simulink model "SimpleTurbine"  (R2023b)
settings: Solver=VariableStepAuto  StartTime=0.0  StopTime=10.0  RelTol=1e-3
undefined symbols (not defined in the file): A_VGS, cp, kap, N, p_in, p_out, R, RH_in, T_in
settings Model: Creator=KOTA-Z  LastModifiedBy=KOTA-Z

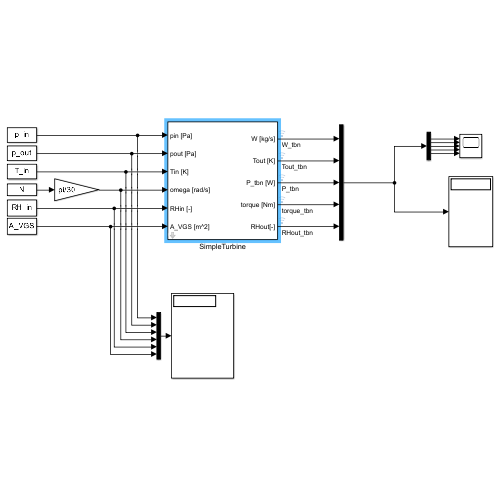
[thumbnail: Simulink's stored preview of the top-level diagram]
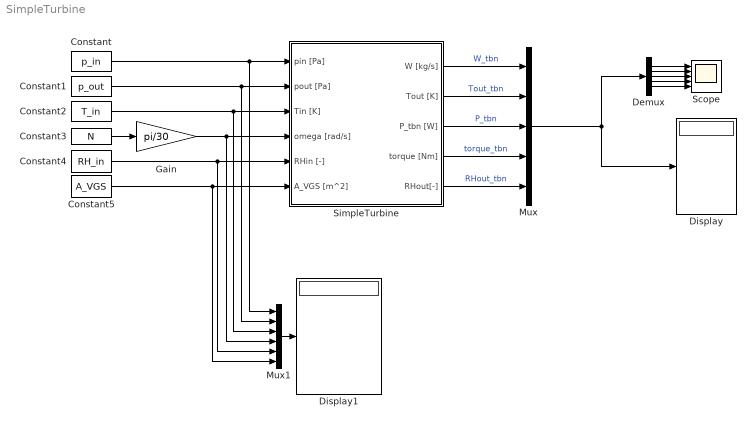
== system SimpleTurbine ==
  Constant : Constant  Value=p_in
  Constant1 : Constant  Value=p_out
  Constant2 : Constant  Value=T_in
  Constant3 : Constant  Value=N
  Constant4 : Constant  Value=RH_in
  Constant5 : Constant  Value=A_VGS
  Demux : Demux  Outputs=5
  Display : Display
  Display1 : Display
  Gain : Gain  Gain=pi/30
  Mux : Mux  Inputs=5
  Mux1 : Mux  Inputs=6
  Scope : Scope  NumInputPorts=5
  SimpleTurbine : Subsystem  mask{eta_is_tbn=0.8, eta_m_tbn=0.98}
      mask prompts: eta_is_tbn "Isentropic efficiency"; eta_m_tbn "Mechanical efficiency"
      mask DialogControl TbnParameters Prompt: Turbine Parameters
  wires:
  Constant2/1 -> Mux1/3, SimpleTurbine/3(Tin [K])
  Constant3/1 -> Gain/1
  Gain/1 -> Mux1/4, SimpleTurbine/4(omega [rad/s])
  Constant4/1 -> Mux1/5, SimpleTurbine/5(RHin [-])
  Constant5/1 -> Mux1/6, SimpleTurbine/6(A_VGS [m^2])
  SimpleTurbine/1(W [kg/s]) -> Mux/1  "W_tbn"
  SimpleTurbine/2(Tout [K]) -> Mux/2  "Tout_tbn"
  SimpleTurbine/3(P_tbn [W]) -> Mux/3  "P_tbn"
  SimpleTurbine/4(torque [Nm]) -> Mux/4  "torque_tbn"
  SimpleTurbine/5(RHout[-]) -> Mux/5  "RHout_tbn"
  Mux/1 -> Demux/1, Display/1
  Demux/1 -> Scope/1
  Demux/2 -> Scope/2
  Demux/3 -> Scope/3
  Demux/4 -> Scope/4
  Demux/5 -> Scope/5
  Mux1/1 -> Display1/1
  Constant/1 -> Mux1/1, SimpleTurbine/1(pin [Pa])
  Constant1/1 -> Mux1/2, SimpleTurbine/2(pout [Pa])

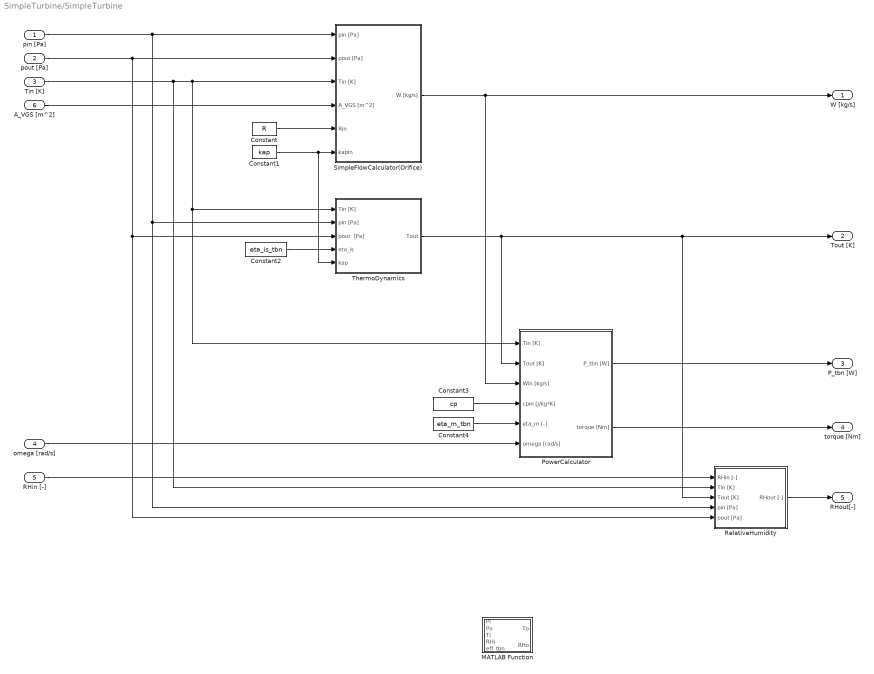
== system SimpleTurbine/SimpleTurbine ==
  pin [Pa] : Inport
  pout [Pa] : Inport  Port=2
  Tin [K] : Inport  Port=3
  omega [rad/s] : Inport  Port=4
  RHin [-] : Inport  Port=5
  A_VGS [m^2] : Inport  Port=6
  Constant : Constant  Value=R
  Constant1 : Constant  Value=kap
  Constant2 : Constant  Value=eta_is_tbn
  Constant3 : Constant  Value=cp
  Constant4 : Constant  Value=eta_m_tbn
  MATLAB Function : MATLAB Function  TreatAsAtomicUnit=on
  PowerCalculator : Subsystem
  RelativeHumidity : Subsystem
  SimpleFlowCalculator(Orifice) : Subsystem
  ThermoDynamics : Subsystem
  W [kg/s] : Outport
  Tout [K] : Outport  Port=2
  P_tbn [W] : Outport  Port=3
  torque [Nm] : Outport  Port=4
  RHout[-] : Outport  Port=5
  wires:
  pin [Pa]/1 -> RelativeHumidity/4(pin [Pa]), ThermoDynamics/2(pin [Pa]), SimpleFlowCalculator(Orifice)/1(pin [Pa])
  Tin [K]/1 -> RelativeHumidity/2(Tin [K]), SimpleFlowCalculator(Orifice)/3(Tin [K]), PowerCalculator/1(Tin [K]), ThermoDynamics/1(Tin [K])
  SimpleFlowCalculator(Orifice)/1(W [kg/s]) -> PowerCalculator/3(Win [kg/s]), W [kg/s]/1
  RHin [-]/1 -> RelativeHumidity/1(RHin [-])
  pout [Pa]/1 -> SimpleFlowCalculator(Orifice)/2(pout [Pa]), RelativeHumidity/5(pout [Pa]), ThermoDynamics/3(pout  [Pa])
  RelativeHumidity/1(RHout [-]) -> RHout[-]/1
  PowerCalculator/1(P_tbn [W]) -> P_tbn [W]/1
  Constant/1 -> SimpleFlowCalculator(Orifice)/5(Rin)
  Constant1/1 -> ThermoDynamics/5(kap), SimpleFlowCalculator(Orifice)/6(kapin)
  Constant2/1 -> ThermoDynamics/4(eta_is)
  Constant3/1 -> PowerCalculator/4(cpin [J/kg*K])
  Constant4/1 -> PowerCalculator/5(eta_m [-])
  omega [rad/s]/1 -> PowerCalculator/6(omega [rad/s])
  PowerCalculator/2(torque [Nm]) -> torque [Nm]/1
  A_VGS [m^2]/1 -> SimpleFlowCalculator(Orifice)/4(A_VGS [m^2])
  ThermoDynamics/1(Tout) -> Tout [K]/1, RelativeHumidity/3(Tout [K]), PowerCalculator/2(Tout [K])

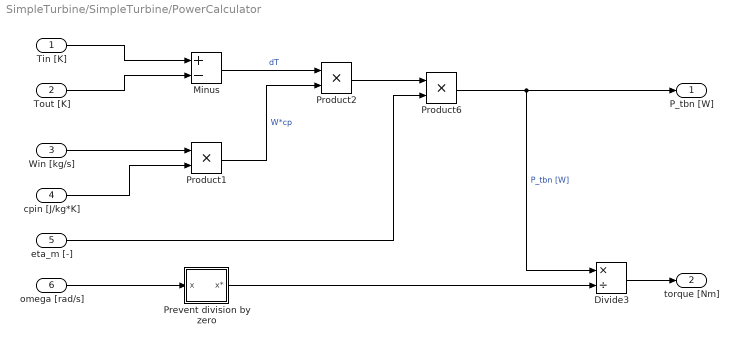
== system SimpleTurbine/SimpleTurbine/PowerCalculator ==
  Tin [K] : Inport
  Tout [K] : Inport  Port=2
  Win [kg/s] : Inport  Port=3
  cpin [J/kg*K] : Inport  Port=4
  eta_m [-] : Inport  Port=5
  omega [rad/s] : Inport  Port=6
  Divide3 : Product  Inputs=*/
  Minus : Sum  Inputs=+-
  Prevent division by zero : Subsystem
  Product1 : Product
  Product2 : Product
  Product6 : Product
  P_tbn [W] : Outport
  torque [Nm] : Outport  Port=2
  wires:
  Tout [K]/1 -> Minus/2
  Tin [K]/1 -> Minus/1
  Minus/1 -> Product2/1  "dT"
  Win [kg/s]/1 -> Product1/1
  cpin [J/kg*K]/1 -> Product1/2
  Product1/1 -> Product2/2  "W*cp"
  Product2/1 -> Product6/1
  eta_m [-]/1 -> Product6/2
  omega [rad/s]/1 -> Prevent division by zero/1(x)
  Divide3/1 -> torque [Nm]/1
  Product6/1 -> P_tbn [W]/1, Divide3/1  "P_tbn [W]"
  Prevent division by zero/1(x*) -> Divide3/2

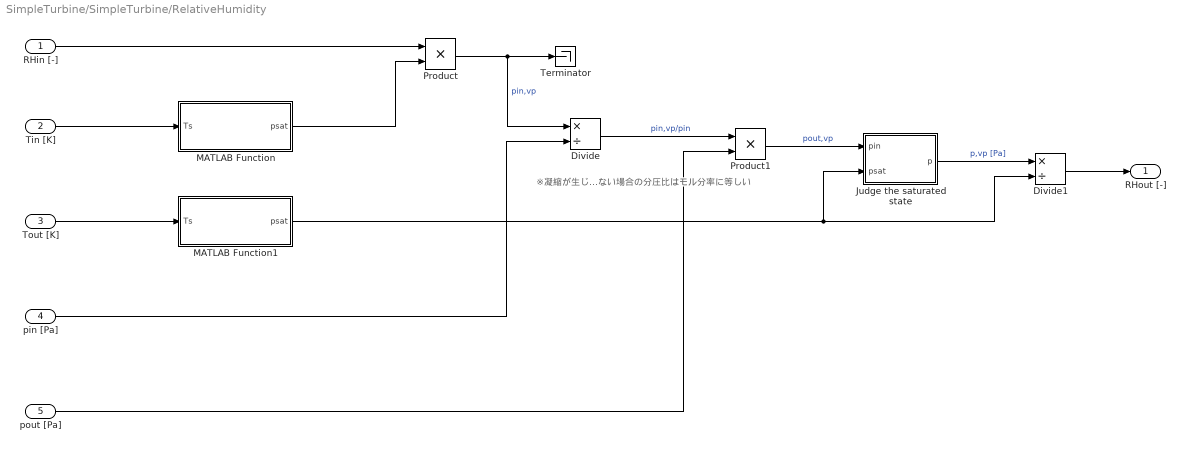
== system SimpleTurbine/SimpleTurbine/RelativeHumidity ==
  note: ※凝縮が生じない場合の分圧比はモル分率に等しい
  RHin [-] : Inport
  Tin [K] : Inport  Port=2
  Tout [K] : Inport  Port=3
  pin [Pa] : Inport  Port=4
  pout [Pa] : Inport  Port=5
  Divide : Product  Inputs=*/
  Divide1 : Product  Inputs=*/
  Judge the saturated state : MATLAB Function  TreatAsAtomicUnit=on
  MATLAB Function : MATLAB Function  TreatAsAtomicUnit=on
  MATLAB Function1 : MATLAB Function  TreatAsAtomicUnit=on
  Product : Product
  Product1 : Product
  Terminator : Terminator
  RHout [-] : Outport
  wires:
  MATLAB Function/1(psat) -> Product/2
  Tin [K]/1 -> MATLAB Function/1(Ts)
  Tout [K]/1 -> MATLAB Function1/1(Ts)
  RHin [-]/1 -> Product/1
  Product/1 -> Terminator/1, Divide/1  "pin,vp"
  pin [Pa]/1 -> Divide/2
  Divide/1 -> Product1/1  "pin,vp/pin"
  pout [Pa]/1 -> Product1/2
  Product1/1 -> Judge the saturated state/1(pin)  "pout,vp"
  MATLAB Function1/1(psat) -> Divide1/2, Judge the saturated state/2(psat)
  Divide1/1 -> RHout [-]/1
  Judge the saturated state/1(p) -> Divide1/1  "p,vp [Pa]"

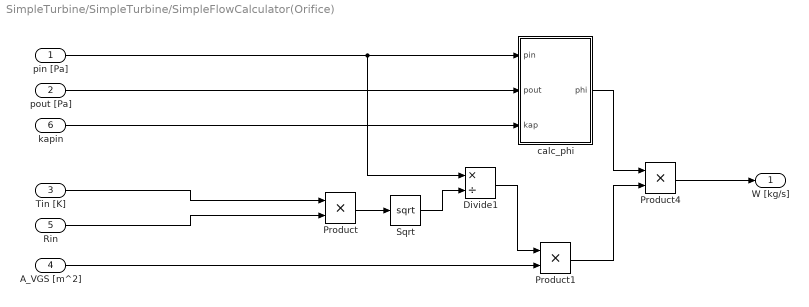
== system SimpleTurbine/SimpleTurbine/SimpleFlowCalculator(Orifice) ==
  pin [Pa] : Inport
  pout [Pa] : Inport  Port=2
  Tin [K] : Inport  Port=3
  A_VGS [m^2] : Inport  Port=4
  Rin : Inport  Port=5
  kapin : Inport  Port=6
  Divide1 : Product  Inputs=*/
  Product : Product
  Product1 : Product
  Product4 : Product
  Sqrt : Sqrt
  calc_phi : MATLAB Function  TreatAsAtomicUnit=on
  W [kg/s] : Outport
  wires:
  pin [Pa]/1 -> Divide1/1, calc_phi/1(pin)
  Divide1/1 -> Product1/1
  Product/1 -> Sqrt/1
  Product4/1 -> W [kg/s]/1
  calc_phi/1(phi) -> Product4/1
  A_VGS [m^2]/1 -> Product1/2
  Tin [K]/1 -> Product/1
  Sqrt/1 -> Divide1/2
  Rin/1 -> Product/2
  Product1/1 -> Product4/2
  pout [Pa]/1 -> calc_phi/2(pout)
  kapin/1 -> calc_phi/3(kap)

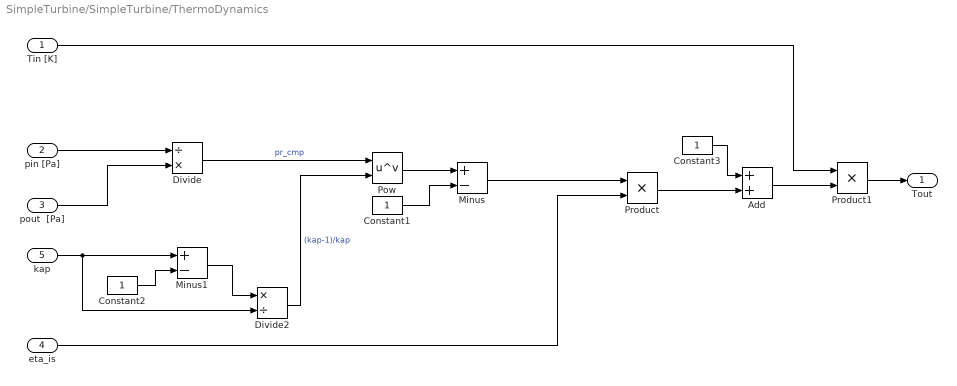
== system SimpleTurbine/SimpleTurbine/ThermoDynamics ==
  Tin [K] : Inport
  pin [Pa] : Inport  Port=2
  pout  [Pa] : Inport  Port=3
  eta_is : Inport  Port=4
  kap : Inport  Port=5
  Add : Sum
  Constant1 : Constant
  Constant2 : Constant
  Constant3 : Constant
  Divide : Product  Inputs=/*
  Divide2 : Product  Inputs=*/
  Minus : Sum  Inputs=+-
  Minus1 : Sum  Inputs=+-
  Pow : Math  Operator=pow  RndMeth=Zero
  Product : Product
  Product1 : Product
  Tout : Outport
  wires:
  Minus/1 -> Product/1
  Divide2/1 -> Pow/2  "(kap-1)/kap"
  Add/1 -> Product1/2
  Constant1/1 -> Minus/2
  Divide/1 -> Pow/1  "pr_cmp"
  Pow/1 -> Minus/1
  Product/1 -> Add/2
  Tin [K]/1 -> Product1/1
  Constant3/1 -> Add/1
  eta_is/1 -> Product/2
  pin [Pa]/1 -> Divide/1
  Product1/1 -> Tout/1
  pout  [Pa]/1 -> Divide/2
  Constant2/1 -> Minus1/2
  kap/1 -> Divide2/2, Minus1/1
  Minus1/1 -> Divide2/1

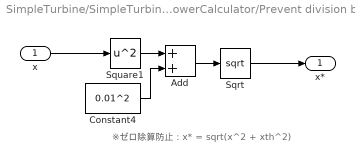
== system SimpleTurbine/SimpleTurbine/PowerCalculator/Prevent division by zero ==
  note: ※ゼロ除算防止 : x* = sqrt(x^2 + xth^2)
  x : Inport
  Add : Sum
  Constant4 : Constant  Value=0.01^2
  Sqrt : Sqrt
  Square1 : Math  Operator=square
  x* : Outport
  wires:
  Constant4/1 -> Add/2
  Square1/1 -> Add/1
  x/1 -> Square1/1
  Add/1 -> Sqrt/1
  Sqrt/1 -> x*/1

== matlab function SimpleTurbine/RelativeHumidity/MATLAB Function ==
  data: Ts input; psat output
function psat = sat_vp_pressure(Ts)
    P_CONVERT = 0.001;
    C1 = -5.6745359e3;
    C2 = 6.3925247;
    C3 = -9.6778430e-3;
    C4 = 6.2215701e-7;
    C5 = 2.0747825e-9;
    C6 = -9.4840240e-13;
    C7 = 4.1635019;
    N1 = 0.11670521452767e4;
    N2 = -0.72421316703206e6;
    N3 = -0.17073846940092e2;
    N4 = 0.12020824702470e5;
    N5 = -0.32325550322333e7;
    N6 = 0.14915108613530e2;
    N7 = -0.4823265731591e4;
    N8 = 0.40511340542057e6;
    N9 = -0.23855557567849e0;
    N10 = 0.65017534844798e3;
    
    if Ts < 273.15+0.01
        % -100~0.01C//三重点を計算以下は wexler-hyland のシミュレーションプログラム式
        psat = exp(C1 / Ts + C2 + C3 * Ts + C4 * Ts^2 + C5 * Ts^3 + C6 * Ts^4 + C7 * log(Ts)) * P_CONVERT;
    else
        %　~647.096K//臨界温度まで一定とするは IAPWS-IF97 実用国際状態式
        alpha = Ts + N9 / (Ts - N10);
        a2 = alpha * alpha;
        A = a2 + N1 * alpha + N2;
        B = N3 * a2 + N4 * alpha + N5;
        C = N6 * a2 + N7 * alpha + N8;
        psat = (2 * C / (-B + (B * B - 4 * A * C)^0.5))^4 / P_CONVERT;
    end 
    psat = psat*1000; %kPa to Pa
end

== matlab function SimpleTurbine/SimpleFlowCalculator(Orifice)/calc_phi ==
  data: pin input; phi output; pout input; kap input
function phi = fcn(pin,pout,kap)
    pr = pout/pin;
    p_cr = (2/(kap+1))^(kap/(kap-1))*pin;
    % Judge critical pressure
    if pout < p_cr
        tmp_phi = sqrt(kap*(2/(kap+1))^((kap+1)/(kap-1)));
    else
        % Prevent to become minus values
        a = 1-pr^((kap-1)/kap);
        %if a < 0
        %    a = 0;
        %end
        tmp_phi = pr^(1/kap)*sqrt(2*kap/(kap-1)*(a));
    end
    phi = tmp_phi;
end

== matlab function SimpleTurbine/RelativeHumidity/MATLAB Function1 ==
  data: Ts input; psat output
function psat = sat_vp_pressure(Ts)
    P_CONVERT = 0.001;
    C1 = -5.6745359e3;
    C2 = 6.3925247;
    C3 = -9.6778430e-3;
    C4 = 6.2215701e-7;
    C5 = 2.0747825e-9;
    C6 = -9.4840240e-13;
    C7 = 4.1635019;
    N1 = 0.11670521452767e4;
    N2 = -0.72421316703206e6;
    N3 = -0.17073846940092e2;
    N4 = 0.12020824702470e5;
    N5 = -0.32325550322333e7;
    N6 = 0.14915108613530e2;
    N7 = -0.4823265731591e4;
    N8 = 0.40511340542057e6;
    N9 = -0.23855557567849e0;
    N10 = 0.65017534844798e3;
    
    if Ts < 273.15+0.01
        % -100~0.01C//三重点を計算以下は wexler-hyland のシミュレーションプログラム式
        psat = exp(C1 / Ts + C2 + C3 * Ts + C4 * Ts^2 + C5 * Ts^3 + C6 * Ts^4 + C7 * log(Ts)) * P_CONVERT;
    else
        %　~647.096K//臨界温度まで一定とするは IAPWS-IF97 実用国際状態式
        alpha = Ts + N9 / (Ts - N10);
        a2 = alpha * alpha;
        A = a2 + N1 * alpha + N2;
        B = N3 * a2 + N4 * alpha + N5;
        C = N6 * a2 + N7 * alpha + N8;
        psat = (2 * C / (-B + (B * B - 4 * A * C)^0.5))^4 / P_CONVERT;
    end 
    psat = psat*1000; %kPa to Pa
end

== matlab function SimpleTurbine/RelativeHumidity/Judge the saturated state ==
  data: pin input; p output; psat input
function p = fcn(pin,psat)
    if pin < psat
        p = pin;
    else
        p = psat;  
    end
end

== matlab function SimpleTurbine/MATLAB Function ==
  data: Pi input; To output; Po input; Ti input; RHi input; eff_tbn input; RHo output
function [To,RHo] = fcn(Pi,Po,Ti,RHi,eff_tbn)

% Calc moist air property
Pwsi = calc_sat_pressure(Ti);   % kPa
Pwi = RHi/100*Pwsi;             % kPa
Wi = 0.62198*Pwi/(Pi-Pwi);      % kg/kg

% calc adiabatic expansion
To_dry = Ti - eff_tbn*(Ti+273.15)*(1-(Pi/Po)^(-(1.4-1)/1.4));
ho_dry = calc_entalpy_air(To_dry, 1.005, 1.805, Wi, 2501.0);

% 凝縮ジャッジ
Pwo = Pwi/Pi*Po;
Pwso = calc_sat_pressure(To_dry);

if Pwo > Pwso
    % disp("凝縮！");
    % Solve turbine outlet temperature by Newton–Raphson method
    % Solver setting
    iteration = 0;
    delta = 1e-10;
    error_min = 1e-5;
    error = 1;
    max_iteration = 999;
    % Initial state
    To = To_dry;
    RHo = 1;
    
    while error > error_min && iteration < max_iteration
        Pwso = calc_sat_pressure(To);
        Wo = 0.62198*Pwso/(Po-Pwso);
        ho = calc_entalpy_mix(To, 1.005, 1.805, 4.186, Wi, Wo, 2501.0);
        fn = ho_dry - ho;
        Pwso_delta = calc_sat_pressure(To+delta);
        Wo_delta = 0.62198*Pwso_delta/(Po-Pwso_delta);
        ho_delta = calc_entalpy_mix(To+delta, 1.005, 1.805, 4.186, Wi, Wo, 2501.0);
        fn_delta = ho_dry - ho_delta;
        df = (fn_delta-fn)/delta;
        df2 = fn/df;
        To = To - 0.1 * fn/((fn_delta-fn)/delta);
        error = abs(ho_dry - calc_entalpy_mix(To, 1.005, 1.805, 4.186, Wi, Wo, 2501.0));
        iteration = iteration + 1;
    end
else
    To = To_dry;
    RHo = Pwo/Pwso;
end

end

function F = calc_sat_pressure(Ts)
    P_CONVERT = 0.001;
    C1 = -5.6745359e3;
    C2 = 6.3925247;
    C3 = -9.6778430e-3;
    C4 = 6.2215701e-7;
    C5 = 2.0747825e-9;
    C6 = -9.4840240e-13;
    C7 = 4.1635019;
    N1 = 0.11670521452767e4;
    N2 = -0.72421316703206e6;
    N3 = -0.17073846940092e2;
    N4 = 0.12020824702470e5;
    N5 = -0.32325550322333e7;
    N6 = 0.14915108613530e2;
    N7 = -0.4823265731591e4;
    N8 = 0.40511340542057e6;
    N9 = -0.23855557567849e0;
    N10 = 0.65017534844798e3;
    Ts_K = Ts + 273.15;
    
    if Ts < 0.01
        % -100~0.01C//三重点を計算以下は wexler-hyland のシミュレーションプログラム式
        F = exp(C1 / Ts_K + C2 + C3 * Ts_K + C4 * Ts_K^2 + C5 * Ts_K^3 + C6 * Ts_K^4 + C7 * log(Ts_K)) * P_CONVERT;
    else
        %　~647.096K//臨界温度まで一定とするは IAPWS-IF97 実用国際状態式
        alpha = Ts_K + N9 / (Ts_K - N10);
        a2 = alpha * alpha;
        A = a2 + N1 * alpha + N2;
        B = N3 * a2 + N4 * alpha + N5;
        C = N6 * a2 + N7 * alpha + N8;
        F = (2 * C / (-B + (B * B - 4 * A * C)^0.5))^4 / P_CONVERT;
    end 
end

function F = calc_entalpy_air(T,Cpa,Cpv,W,hg0)
    T_K = T+273.15;
    F = Cpa*T_K+W*(Cpv*T_K+hg0);
end

function F = calc_entalpy_mix(T,Cpa,Cpv,Cpw,W1,W2,hg0)
    T_K = T+273.15;
    F = Cpa*T_K+W2*(Cpv*T_K+hg0)+(W1-W2)*Cpw*T_K;
end
